simulink library "gradient_ul"  (R2018a)
settings: Solver=VariableStepAuto  StartTime=0.0  StopTime=10.0  RelTol=1e-3
settings Model: Creator=mitch  LastModifiedBy=mitch

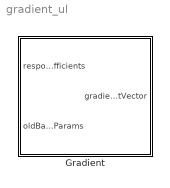
== system gradient_ul ==
  Gradient : Subsystem

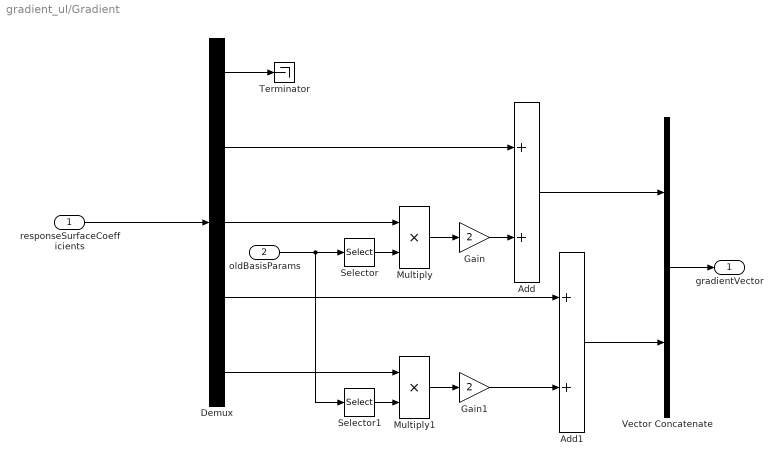
== system gradient_ul/Gradient ==
  responseSurfaceCoefficients : Inport
  oldBasisParams : Inport  Port=2
  Add : Sum
  Add1 : Sum
  Demux : Demux  Outputs=5
  Gain : Gain  Gain=2
  Gain1 : Gain  Gain=2
  Multiply : Product
  Multiply1 : Product
  Selector : Selector  InputPortWidth=2  IndexOptions=Index vector (dialog)  Indices=1  OutputSizes=1
  Selector1 : Selector  InputPortWidth=2  IndexOptions=Index vector (dialog)  Indices=2  OutputSizes=1
  Terminator : Terminator
  Vector Concatenate : Concatenate
  gradientVector : Outport
  wires:
  Vector Concatenate/1 -> gradientVector/1
  Demux/4 -> Add1/1
  Selector1/1 -> Multiply1/2
  Demux/3 -> Multiply/1
  Gain1/1 -> Add1/2
  Demux/5 -> Multiply1/1
  responseSurfaceCoefficients/1 -> Demux/1
  Demux/1 -> Terminator/1
  Multiply/1 -> Gain/1
  Multiply1/1 -> Gain1/1
  Add1/1 -> Vector Concatenate/2
  Gain/1 -> Add/2
  Selector/1 -> Multiply/2
  Demux/2 -> Add/1
  oldBasisParams/1 -> Selector/1, Selector1/1
  Add/1 -> Vector Concatenate/1
